simulink model "regulator_z_calkowaniem"  (R2022a)
settings: Solver=VariableStepAuto  StartTime=0.0  StopTime=50  RelTol=1e-3
values from neighbouring files (symbols this model uses):
  K = acker(Ar, Br, [sb sb sb sb])    [dane.m]
  mnoznik = 1.30    (= 1.3)    [dane.m]
settings Model: Creator=danie  LastModifiedBy=danie

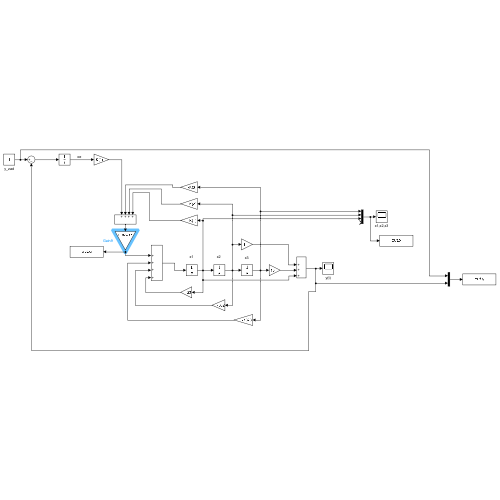
[thumbnail: Simulink's stored preview of the top-level diagram]
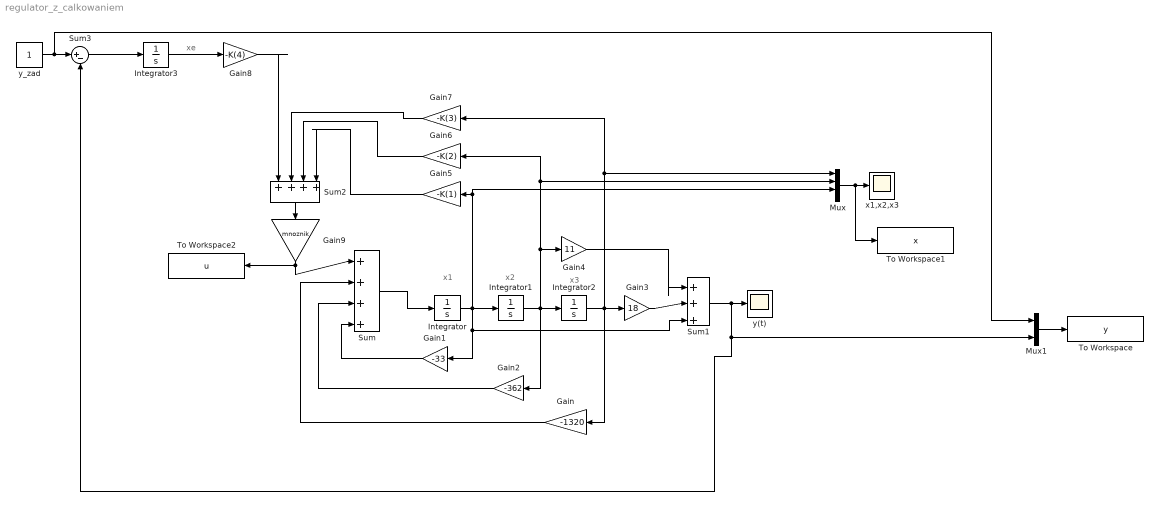
== system regulator_z_calkowaniem ==
  note: xe
  note: x1
  note: x3
  note: x2
  Gain : Gain  Gain=-1320
  Gain1 : Gain  Gain=-33
  Gain2 : Gain  Gain=-362
  Gain3 : Gain  Gain=18
  Gain4 : Gain  Gain=11
  Gain5 : Gain  Gain=-K(1)
  Gain6 : Gain  Gain=-K(2)
  Gain7 : Gain  Gain=-K(3)
  Gain8 : Gain  Gain=-K(4)
  Gain9 : Gain  Gain=mnoznik
  Integrator{,1..3} (4 alike) : Integrator
  Mux : Mux
  Mux1 : Mux  Inputs=2
  Sum : Sum  Inputs=|++++
  Sum1 : Sum  Inputs=|+++
  Sum2 : Sum  Inputs=|++++
  Sum3 : Sum  Inputs=|+-
  To Workspace : ToWorkspace  VariableName=y  SaveFormat=Structure With Time  SampleTime=-1
  To Workspace1 : ToWorkspace  VariableName=x  SaveFormat=Structure With Time  SampleTime=-1
  To Workspace2 : ToWorkspace  VariableName=u  SaveFormat=Structure With Time  SampleTime=-1
  x1,x2,x3 : Scope
  y(t) : Scope
  y_zad : Constant
  wires:
  Mux/1 -> To Workspace1/1, x1,x2,x3/1
  Sum1/1 -> Mux1/2, Sum3/2, y(t)/1
  Integrator2/1 -> Gain7/1, Mux/1, Gain/1, Gain3/1
  Gain1/1 -> Sum/4
  Gain3/1 -> Sum1/2
  Gain2/1 -> Sum/3
  Sum/1 -> Integrator/1
  Integrator/1 -> Sum1/3, Gain1/1, Integrator1/1, Mux/3, Gain5/1
  Gain4/1 -> Sum1/1
  Integrator1/1 -> Gain4/1, Gain6/1, Mux/2, Gain2/1, Integrator2/1
  Gain/1 -> Sum/2
  y_zad/1 -> Mux1/1, Sum3/1
  Sum3/1 -> Integrator3/1
  Gain7/1 -> Sum2/2
  Gain6/1 -> Sum2/3
  Gain5/1 -> Sum2/4
  Integrator3/1 -> Gain8/1
  Gain8/1 -> Sum2/1
  Mux1/1 -> To Workspace/1
  Sum2/1 -> Gain9/1
  Gain9/1 -> Sum/1, To Workspace2/1
